simulink model "simple_plant_model"  (R2018a)
settings: Solver=VariableStepAuto  StartTime=0.0  StopTime=10.0  RelTol=1e-3
settings Model: Creator=Kim  LastModifiedBy=Kim

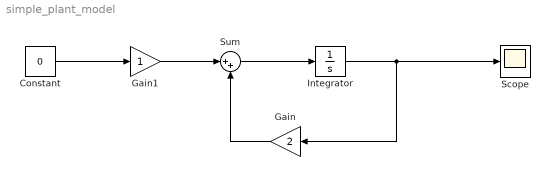
== system simple_plant_model ==
  Constant : Constant  Value=0
  Gain : Gain  Gain=2
  Gain1 : Gain
  Integrator : Integrator  InitialCondition=0.1
  Scope : Scope
  Sum : Sum  Inputs=|++
  wires:
  Sum/1 -> Integrator/1
  Integrator/1 -> Scope/1, Gain/1
  Gain/1 -> Sum/2
  Gain1/1 -> Sum/1
  Constant/1 -> Gain1/1
